simulink model "ObservadorDig"  (R2022b)
settings: Solver=VariableStepAuto  StartTime=0.0  StopTime=10.0  RelTol=1e-3
values from neighbouring files (symbols this model uses):
  A = [-1 -2 ... (first row only)    [ABinvariantes11deJunio.m]    (also in Convertibility.m = [0 1 0  0 0; DivirsoresElementales.m = [1 0 -1; 0 1 0; 0 0 2]; Examen.m = [1 1;0 1]; Examen2.m = [0 0  0 0 0)
  B = [1 ... (first row only)    [ABinvariantes11deJunio.m]    (also in Convertibility.m = [0 0; Examen.m = [1;0]; Examen2.m = [1 0; Sestrella.m = [0;1;0])
  C = [1 0]    [Examen.m]    (also in Sestrella.m = [0 1 0; 0 0 1]; Westrella.m = [0 1 0; 0 0 1])
  D = [2 -3]    [ABinvariantes11deJunio.m]    (also in Examen2.m = [0 0 0 1 0]; V_estrella.m = [0 0 0 1 0]; Westrella.m = [1 0)
  G = P*B    [Westrella.m]
  L = [0 ;0; 1]    [Sestrella.m]    (also in Westrella.m)
settings Model: Creator=raul  LastModifiedBy=raul

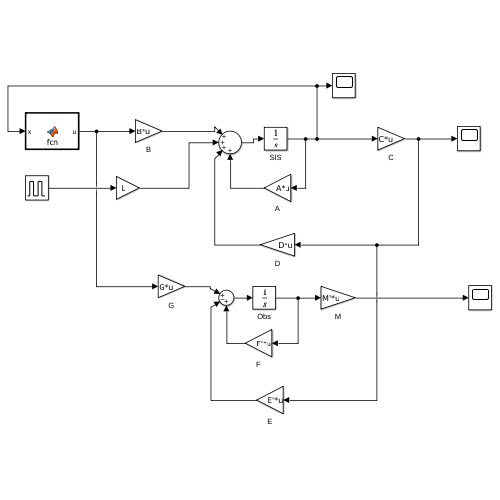
[thumbnail: Simulink's stored preview of the top-level diagram]
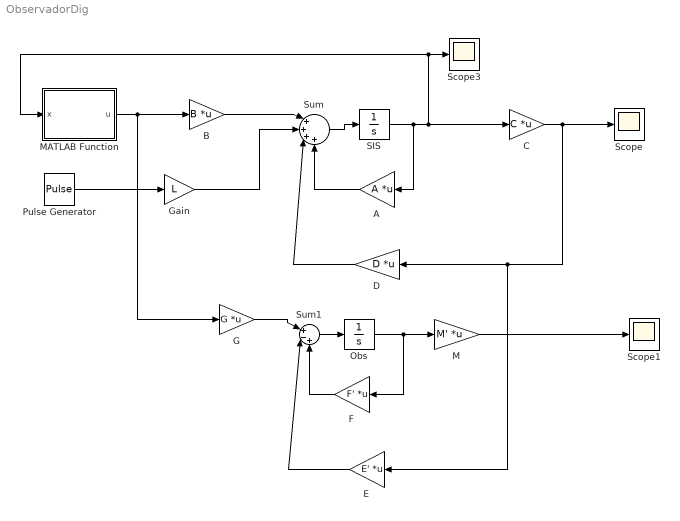
== system ObservadorDig ==
  A : Gain  Gain=A  Multiplication=Matrix(K*u)
  B : Gain  Gain=B  Multiplication=Matrix(K*u)
  C : Gain  Gain=C  Multiplication=Matrix(K*u)
  D : Gain  Gain=D  Multiplication=Matrix(K*u)
  E : Gain  Gain=E'  Multiplication=Matrix(K*u)
  F : Gain  Gain=F'  Multiplication=Matrix(K*u)
  G : Gain  Gain=G  Multiplication=Matrix(K*u)
  Gain : Gain  Gain=L
  M : Gain  Gain=M'  Multiplication=Matrix(K*u)
  MATLAB Function : MATLAB Function  TreatAsAtomicUnit=on
  Obs : Integrator  InitialCondition=[1;1]
  Pulse Generator : DiscretePulseGenerator  PulseType=Time based  Period=10  PulseWidth=5
  SIS : Integrator  InitialCondition=[1;1;1]
  Scope : Scope
  Scope1 : Scope
  Scope3 : Scope
  Sum : Sum  Inputs=|++++
  Sum1 : Sum  Inputs=|+-+
  wires:
  B/1 -> Sum/1
  C/1 -> Scope/1, E/1, D/1
  SIS/1 -> A/1, C/1, Scope3/1, MATLAB Function/1(x)
  Sum/1 -> SIS/1
  Obs/1 -> F/1, M/1
  M/1 -> Scope1/1
  G/1 -> Sum1/1
  Sum1/1 -> Obs/1
  F/1 -> Sum1/3
  E/1 -> Sum1/2
  A/1 -> Sum/4
  D/1 -> Sum/3
  Gain/1 -> Sum/2
  Pulse Generator/1 -> Gain/1
  MATLAB Function/1(u) -> G/1, B/1

== matlab function ObservadorDig/MATLAB Function ==
  data: x input; u output
function u = fcn(x)
R=[20 4 0];
u = -R*x;
